simulink model "test_export_check"  (R2026a)
settings: Solver=FixedStepAuto
values from neighbouring files (symbols this model uses):
  net = coder.loadDeepLearningNetwork('soc_compressed_opt5.mat', 'bestNet')    [predict_soc_compressed_opt5.m]    (also in predict_soc_opt5_direct.m = coder.loadDeepLearningNetwork('soc_basenet_opt5.mat', 'baseN)
libraries: dlconvfclib x2, dlsequencelib x2, dlactivationlib x1
settings Model: Creator=arkadiyturevskiy  LastModifiedBy=arkadiyturevskiy
settings RTWCC: SystemTargetFile=ert.tlc  Description=Embedded Coder
settings ERTTargetCC: GenerateSampleERTMain=on

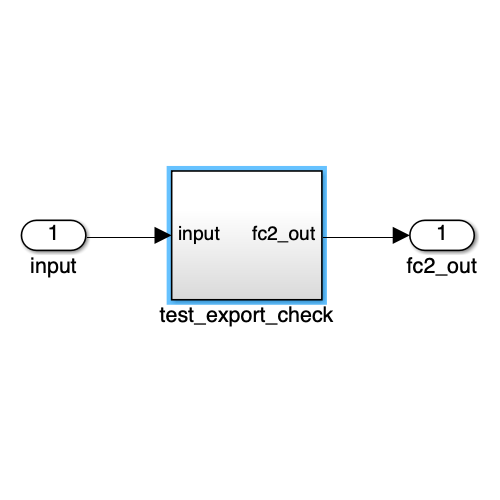
[thumbnail: Simulink's stored preview of the top-level diagram]
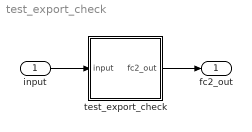
== system test_export_check ==
  input : Inport  PortDimensions="[5  1]"
  test_export_check : Subsystem
  fc2_out : Outport
  wires:
  test_export_check/1(fc2_out) -> fc2_out/1
  input/1 -> test_export_check/1(input)

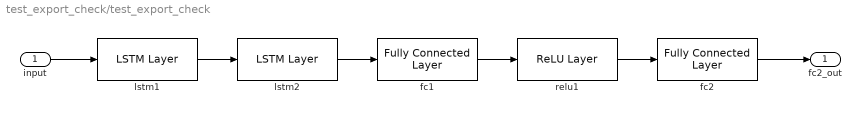
== system test_export_check/test_export_check ==
  input : Inport  PortDimensions="[5  1]"
  fc1 : dlconvfclib/Fully Connected Layer  Layer=net.Layers(4)  OutMin=[]  OutMax=[]  WeightsDataTypeStr=Inherit: Inherit via back propagation  WeightsMin=[]  WeightsMax=[]  BiasDataTypeStr=Inherit: Inherit via back propagation  BiasMin=[]  BiasMax=[]  AccumMin=[]  AccumMax=[]  InternalRndMeth=Floor  InternalSaturateOnIntegerOverflow=off  SampleTime=-1
      settings: DataFormat=C
  fc2 : dlconvfclib/Fully Connected Layer  Layer=net.Layers(6)  OutMin=[]  OutMax=[]  WeightsDataTypeStr=Inherit: Inherit via back propagation  WeightsMin=[]  WeightsMax=[]  BiasDataTypeStr=Inherit: Inherit via back propagation  BiasMin=[]  BiasMax=[]  AccumMin=[]  AccumMax=[]  InternalRndMeth=Floor  InternalSaturateOnIntegerOverflow=off  SampleTime=-1
      settings: DataFormat=C
  lstm1 : dlsequencelib/LSTM Layer  Layer=net.Layers(2)  Stateful=on  ApproximationMethod=None  OutMin=[]  OutMax=[]  InputWeightsDataTypeStr=Inherit: Inherit via back propagation  InputWeightsMin=[]  InputWeightsMax=[]  RecurrentWeightsDataTypeStr=Inherit: Inherit via back propagation  RecurrentWeightsMin=[]  RecurrentWeightsMax=[]  BiasDataTypeStr=Inherit: Inherit via back propagation  BiasMin=[]  BiasMax=[]  InitialCellStateDataTypeStr=Inherit: Inherit via back propagation  InitialCellStateMin=[]  InitialCellStateMax=[]  CellStateMin=[]  CellStateMax=[]  InitialHiddenStateDataTypeStr=Inherit: Inherit via back propagation  InitialHiddenStateMin=[]  InitialHiddenStateMax=[]  HiddenStateMin=[]  HiddenStateMax=[]  InputWeightsMatrixMultiplyOutMin=[]  InputWeightsMatrixMultiplyOutMax=[]  RecurrentWeightsMatrixMultiplyOutMin=[]  RecurrentWeightsMatrixMultiplyOutMax=[]  LinearGateAddOutMin=[]  LinearGateAddOutMax=[]  CellStateProductOutMin=[]  CellStateProductOutMax=[]  SampleTime=-1
      settings: DataFormat=CT
  lstm2 : dlsequencelib/LSTM Layer  Layer=net.Layers(3)  Stateful=on  ApproximationMethod=None  OutMin=[]  OutMax=[]  InputWeightsDataTypeStr=Inherit: Inherit via back propagation  InputWeightsMin=[]  InputWeightsMax=[]  RecurrentWeightsDataTypeStr=Inherit: Inherit via back propagation  RecurrentWeightsMin=[]  RecurrentWeightsMax=[]  BiasDataTypeStr=Inherit: Inherit via back propagation  BiasMin=[]  BiasMax=[]  InitialCellStateDataTypeStr=Inherit: Inherit via back propagation  InitialCellStateMin=[]  InitialCellStateMax=[]  CellStateMin=[]  CellStateMax=[]  InitialHiddenStateDataTypeStr=Inherit: Inherit via back propagation  InitialHiddenStateMin=[]  InitialHiddenStateMax=[]  HiddenStateMin=[]  HiddenStateMax=[]  InputWeightsMatrixMultiplyOutMin=[]  InputWeightsMatrixMultiplyOutMax=[]  RecurrentWeightsMatrixMultiplyOutMin=[]  RecurrentWeightsMatrixMultiplyOutMax=[]  LinearGateAddOutMin=[]  LinearGateAddOutMax=[]  CellStateProductOutMin=[]  CellStateProductOutMax=[]  SampleTime=-1
      settings: DataFormat=CT
  relu1 : dlactivationlib/ReLU Layer  OutMin=[]  OutMax=[]  SampleTime=-1
  fc2_out : Outport
  wires:
  relu1/1 -> fc2/1
  lstm2/1 -> fc1/1
  lstm1/1 -> lstm2/1
  input/1 -> lstm1/1
  fc2/1 -> fc2_out/1
  fc1/1 -> relu1/1
